simulink subsystem "E_Reg_Valves"  (R2025a)
settings: Solver=VariableStepAuto  StartTime=0.0  StopTime=10.0  RelTol=1e-3
undefined symbols (not defined in the file): EREG_command_sample_time_s, EREG_gear_ratio, EREG_normalised_area_table, EREG_servo_angle_max_deg, EREG_servo_rate_degps, EREG_valve_angle_breakpoints_deg, EREG_valve_angle_max_deg, EREG_valve_angle_min_deg
libraries: SimscapeFluids_lib x4, nesl_utility x2
settings Model: Creator=Adam  LastModifiedBy=dj23106

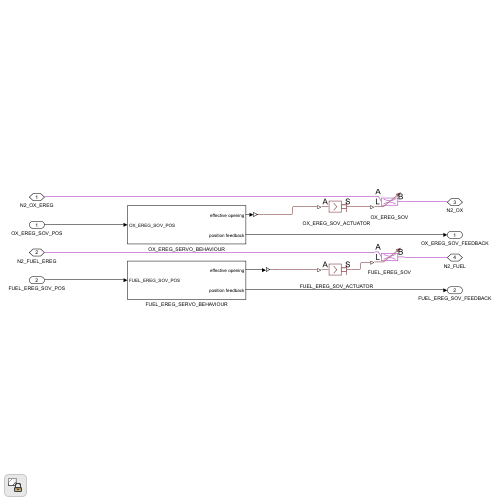
[thumbnail: Simulink's stored preview of the top-level diagram]
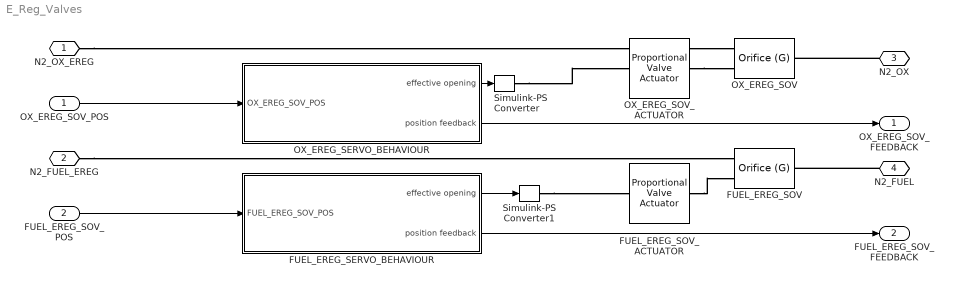
== system E_Reg_Valves ==
  OX_EREG_SOV_POS : Inport
  FUEL_EREG_SOV_POS : Inport  Port=2
  FUEL_EREG_SERVO_BEHAVIOUR : Subsystem
  FUEL_EREG_SOV : SimscapeFluids_lib/Gas/Valves & Orifices/Orifice (G)  orifice_type=foundation.enum.constant_variable.variable  orifice_parameterization=fluids.gas.valves_orifices.enum.OrificeParameterization.Cv  opening_characteristic=fluids.gas.valves_orifices.enum.OpeningCharacteristics.Linear  Cv_constant=4  Cv_max=Cv_max  L_Cv_TLU=0 : 0.2 : 1  Cv_TLU=[1e-06, .8, 1.6, 2.4, 3.2, 4]  xT_Cv=0.7  Kv_constant=3.6  Kv_max=3.6  L_Kv_TLU=0 : 0.2 : 1  Kv_TLU=[1e-06, .72, 1.44, 2.16, 2.88, 3.6]  xT_Kv=0.7  C_constant=12 l/(bar*s)  B_crit_constant=0.3  C_max=12 l/(bar*s)  B_crit_linear=0.3  L_C_TLU=0 : 0.2 : 1  C_TLU=[1e-05, 2.4, 4.8, 7.2, 9.6, 12] l/(bar*s)  B_crit_TLU=0.3 * ones(1, 6)  m=0.5  T_ref_C=293.15 K  rho_ref_C=1.185 kg/m^3  orifice_area_constant=1e-4 m^2  orifice_area_max=1e-4 m^2  L_orifice_area_TLU=0 : 0.2 : 1  orifice_area_TLU=[1e-10, 2e-05, 4e-05, 6e-05, 8e-05, .0001] m^2  Cd=0.64  leakage_fraction=1e-6  smoothing_factor=0.01  B_lam=0.999  area=0.01 m^2
      settings: InternalSimscapePortConfiguration="{\"Bottom\":[],\"Left\":[{\"id\":\"A\",\"label\":\"A\",\"type\":\"foundation.gas.gas\"},{\"id\":\"L\",\"label\":\"L\",\"type\":\"input\"}],\"Right\":[{\"id\":\"B\",\"label\":\"B\",\"type\":\"foundation.gas.gas\"}],\"Top\":[]}"
  FUEL_EREG_SOV_ACTUATOR : SimscapeFluids_lib/Valve Actuators/Proportional Valve Actuator  gain=5e-4 m  time_constant=0.01 s  valve_stroke=0.005 m
      settings: InternalSimscapePortConfiguration="{\"Bottom\":[],\"Left\":[{\"id\":\"A\",\"label\":\"A\",\"type\":\"input\"}],\"Right\":[{\"id\":\"S\",\"label\":\"S\",\"type\":\"output\"}],\"Top\":[]}"
  OX_EREG_SERVO_BEHAVIOUR : Subsystem
  OX_EREG_SOV : SimscapeFluids_lib/Gas/Valves & Orifices/Orifice (G)  orifice_type=foundation.enum.constant_variable.variable  orifice_parameterization=fluids.gas.valves_orifices.enum.OrificeParameterization.Cv  opening_characteristic=fluids.gas.valves_orifices.enum.OpeningCharacteristics.Linear  Cv_constant=4  Cv_max=Cv_max  L_Cv_TLU=0 : 0.2 : 1  Cv_TLU=[1e-06, .8, 1.6, 2.4, 3.2, 4]  xT_Cv=0.7  Kv_constant=3.6  Kv_max=3.6  L_Kv_TLU=0 : 0.2 : 1  Kv_TLU=[1e-06, .72, 1.44, 2.16, 2.88, 3.6]  xT_Kv=0.7  C_constant=12 l/(bar*s)  B_crit_constant=0.3  C_max=12 l/(bar*s)  B_crit_linear=0.3  L_C_TLU=0 : 0.2 : 1  C_TLU=[1e-05, 2.4, 4.8, 7.2, 9.6, 12] l/(bar*s)  B_crit_TLU=0.3 * ones(1, 6)  m=0.5  T_ref_C=293.15 K  rho_ref_C=1.185 kg/m^3  orifice_area_constant=1e-4 m^2  orifice_area_max=1e-4 m^2  L_orifice_area_TLU=0 : 0.2 : 1  orifice_area_TLU=[1e-10, 2e-05, 4e-05, 6e-05, 8e-05, .0001] m^2  Cd=0.64  leakage_fraction=1e-6  smoothing_factor=0.01  B_lam=0.999  area=0.01 m^2
      settings: InternalSimscapePortConfiguration="{\"Bottom\":[],\"Left\":[{\"id\":\"A\",\"label\":\"A\",\"type\":\"foundation.gas.gas\"},{\"id\":\"L\",\"label\":\"L\",\"type\":\"input\"}],\"Right\":[{\"id\":\"B\",\"label\":\"B\",\"type\":\"foundation.gas.gas\"}],\"Top\":[]}"
  OX_EREG_SOV_ACTUATOR : SimscapeFluids_lib/Valve Actuators/Proportional Valve Actuator  gain=5e-4 m  time_constant=0.01 s  valve_stroke=0.005 m
      settings: InternalSimscapePortConfiguration="{\"Bottom\":[],\"Left\":[{\"id\":\"A\",\"label\":\"A\",\"type\":\"input\"}],\"Right\":[{\"id\":\"S\",\"label\":\"S\",\"type\":\"output\"}],\"Top\":[]}"
  Simulink-PS Converter : nesl_utility/Simulink-PS Converter  PhysicalDomain=network_engine_domain  SubClassName=ps_input  LeftPortType=input  RightPortType=output  PseudoPeriodic=off  Frequencies=[]  NoiseDistribution=none  NoiseParameters=[]  Unit=1  AffineConversion=off  FilteringAndDerivatives=provide  SimscapeFilterOrder=1  InputFilterTimeConstant=0.001  UdotUserProvided=0
  Simulink-PS Converter1 : nesl_utility/Simulink-PS Converter  PhysicalDomain=network_engine_domain  SubClassName=ps_input  LeftPortType=input  RightPortType=output  PseudoPeriodic=off  Frequencies=[]  NoiseDistribution=none  NoiseParameters=[]  Unit=1  AffineConversion=off  FilteringAndDerivatives=provide  SimscapeFilterOrder=1  InputFilterTimeConstant=0.001  UdotUserProvided=0
  N2_OX_EREG : PMIOPort  Side=Left
  N2_FUEL_EREG : PMIOPort  Port=2  Side=Left
  N2_OX : PMIOPort  Port=3  Side=Right
  N2_FUEL : PMIOPort  Port=4  Side=Right
  OX_EREG_SOV_FEEDBACK : Outport
  FUEL_EREG_SOV_FEEDBACK : Outport  Port=2
  wires:
  OX_EREG_SOV_POS/1 -> OX_EREG_SERVO_BEHAVIOUR/1(OX_EREG_SOV_POS)
  OX_EREG_SERVO_BEHAVIOUR/1(effective opening) -> Simulink-PS Converter/1
  OX_EREG_SERVO_BEHAVIOUR/2(position feedback) -> OX_EREG_SOV_FEEDBACK/1
  FUEL_EREG_SOV_POS/1 -> FUEL_EREG_SERVO_BEHAVIOUR/1(FUEL_EREG_SOV_POS)
  FUEL_EREG_SERVO_BEHAVIOUR/1(effective opening) -> Simulink-PS Converter1/1
  FUEL_EREG_SERVO_BEHAVIOUR/2(position feedback) -> FUEL_EREG_SOV_FEEDBACK/1
  connections:
  OX_EREG_SOV_ACTUATOR/RConn1 -- OX_EREG_SOV/LConn2
  N2_OX_EREG/RConn1 -- OX_EREG_SOV/LConn1
  N2_OX/RConn1 -- OX_EREG_SOV/RConn1
  FUEL_EREG_SOV_ACTUATOR/RConn1 -- FUEL_EREG_SOV/LConn2
  Simulink-PS Converter1/RConn1 -- FUEL_EREG_SOV_ACTUATOR/LConn1
  N2_FUEL/RConn1 -- FUEL_EREG_SOV/RConn1
  N2_FUEL_EREG/RConn1 -- FUEL_EREG_SOV/LConn1
  Simulink-PS Converter/RConn1 -- OX_EREG_SOV_ACTUATOR/LConn1

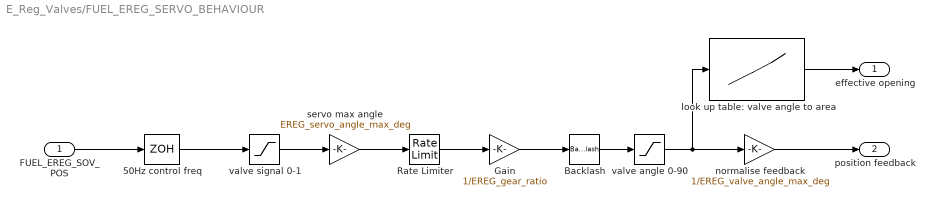
== system E_Reg_Valves/FUEL_EREG_SERVO_BEHAVIOUR ==
  FUEL_EREG_SOV_POS : Inport
  50Hz control freq : ZeroOrderHold  SampleTime=EREG_command_sample_time_s
  Backlash : Backlash  BacklashWidth=EREG_valve_backlash_deg
  Gain : Gain  Gain=1/EREG_gear_ratio
  Rate Limiter : RateLimiter  RisingSlewLimit=EREG_servo_rate_degps  FallingSlewLimit=-EREG_servo_rate_degps  SampleTimeMode=inherited
  look up table: valve angle to area : Lookup_n-D  NumberOfTableDimensions=1  BreakpointsForDimension1=EREG_valve_angle_breakpoints_deg  Table=EREG_normalised_area_table  InternalRulePriority=Speed  RndMeth=Simplest
  normalise feedback : Gain  Gain=1/EREG_valve_angle_max_deg
  servo max angle : Gain  Gain=EREG_servo_angle_max_deg
  valve angle 0-90 : Saturate  UpperLimit=EREG_valve_angle_max_deg  LowerLimit=EREG_valve_angle_min_deg
  valve signal 0-1 : Saturate  UpperLimit=1  LowerLimit=0
  effective opening : Outport
  position feedback : Outport  Port=2
  wires:
  normalise feedback/1 -> position feedback/1
  valve angle 0-90/1 -> normalise feedback/1, look up table: valve angle to area/1
  look up table: valve angle to area/1 -> effective opening/1
  Backlash/1 -> valve angle 0-90/1
  Gain/1 -> Backlash/1
  Rate Limiter/1 -> Gain/1
  servo max angle/1 -> Rate Limiter/1
  valve signal 0-1/1 -> servo max angle/1
  50Hz control freq/1 -> valve signal 0-1/1
  FUEL_EREG_SOV_POS/1 -> 50Hz control freq/1

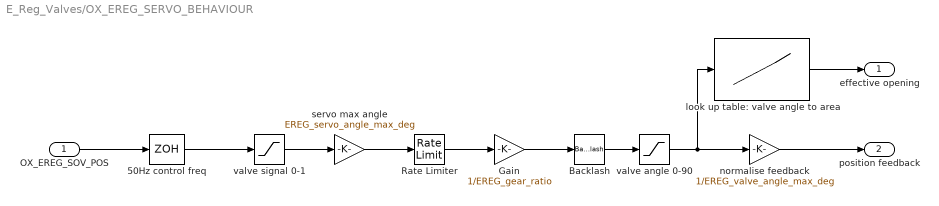
== system E_Reg_Valves/OX_EREG_SERVO_BEHAVIOUR ==
  OX_EREG_SOV_POS : Inport
  50Hz control freq : ZeroOrderHold  SampleTime=EREG_command_sample_time_s
  Backlash : Backlash  BacklashWidth=EREG_valve_backlash_deg
  Gain : Gain  Gain=1/EREG_gear_ratio
  Rate Limiter : RateLimiter  RisingSlewLimit=EREG_servo_rate_degps  FallingSlewLimit=-EREG_servo_rate_degps  SampleTimeMode=inherited
  look up table: valve angle to area : Lookup_n-D  NumberOfTableDimensions=1  BreakpointsForDimension1=EREG_valve_angle_breakpoints_deg  Table=EREG_normalised_area_table  InternalRulePriority=Speed  RndMeth=Simplest
  normalise feedback : Gain  Gain=1/EREG_valve_angle_max_deg
  servo max angle : Gain  Gain=EREG_servo_angle_max_deg
  valve angle 0-90 : Saturate  UpperLimit=EREG_valve_angle_max_deg  LowerLimit=EREG_valve_angle_min_deg
  valve signal 0-1 : Saturate  UpperLimit=1  LowerLimit=0
  effective opening : Outport
  position feedback : Outport  Port=2
  wires:
  normalise feedback/1 -> position feedback/1
  valve angle 0-90/1 -> normalise feedback/1, look up table: valve angle to area/1
  look up table: valve angle to area/1 -> effective opening/1
  Backlash/1 -> valve angle 0-90/1
  Gain/1 -> Backlash/1
  Rate Limiter/1 -> Gain/1
  servo max angle/1 -> Rate Limiter/1
  valve signal 0-1/1 -> servo max angle/1
  50Hz control freq/1 -> valve signal 0-1/1
  OX_EREG_SOV_POS/1 -> 50Hz control freq/1
